simulink model "IndicatorModule"  (R2025b)
settings: Solver=VariableStepAuto  StartTime=0.0  StopTime=10.0  RelTol=1e-3
settings Model: Creator=sinch  LastModifiedBy=sinch
settings OptimizationCC: DefaultParameterBehavior=Inlined  EnhancedBackFolding=on  PassReuseOutputArgsAs=Individual arguments  ZeroExternalMemoryAtStartup=off  ZeroInternalMemoryAtStartup=off  OptimizeBlockOrder=speed  DifferentSizesBufferReuse=on  OptimizationCustomize=off  EfficientTunableParamExpr=on
settings DebuggingCC: ParameterTunabilityLossMsg=error
settings SFSimCC: MATLABDynamicMemAlloc=off
settings RTWCC: SystemTargetFile=ert.tlc  TemplateMakefile=ert_default_tmf  Description=Embedded Coder
settings CodeAppCC: ForceParamTrailComments=on  IgnoreCustomStorageClasses=off  OperatorAnnotations=on  SimulinkDataObjDesc=on  SFDataObjDesc=on  InsertBlockDesc=on
settings ERTTargetCC: ERTCustomFileTemplate=example_file_process.tlc  TargetLangStandard=C99 (ISO)  GenerateSampleERTMain=on

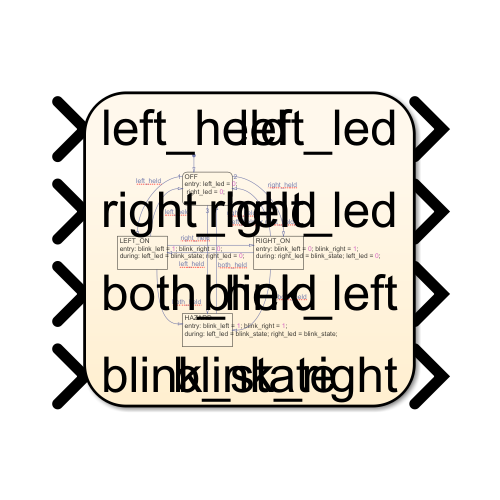
[thumbnail: Simulink's stored preview of the top-level diagram]
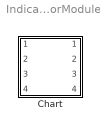
== system IndicatorModule ==
  Chart : Stateflow chart  TreatAsAtomicUnit=on

== stateflow chart IndicatorModule/Chart ==
  state OFF
    entry: left_led = 0;
    right_led = 0;
  state LEFT_ON [group]
    entry: blink_left = 1; blink_right = 0;
    during: left_led = blink_state; right_led = 0;
  state RIGHT_ON [group]
    entry: blink_left = 0; blink_right = 1;
    during: right_led = blink_state; left_led = 0;
  state HAZARD [group]
    entry: blink_left = 1; blink_right = 1;
    during: left_led = blink_state; right_led = blink_state;
  (default) -> OFF
  OFF -> LEFT_ON [order 1] : left_held
  OFF -> RIGHT_ON [order 2] : right_held
  LEFT_ON -> OFF [order 4294967295] : left_held
  RIGHT_ON -> OFF [order 4294967295] : right_held
  OFF -> HAZARD [order 3] : both_held
  HAZARD -> OFF : [left_held or right_held]
  LEFT_ON -> RIGHT_ON [order 4294967295] : right_held
  RIGHT_ON -> LEFT_ON [order 4294967295] : left_held
  LEFT_ON -> HAZARD [order 4294967295] : both_held
  RIGHT_ON -> HAZARD [order 4294967295] : both_held
  data: left_held input boolean; right_held input boolean; both_held input boolean; blink_state input boolean; left_led output boolean; right_led output boolean; blink_left output boolean; blink_right output boolean
